simulink model "orbitCon"  (R2015b)
settings: Solver=VariableStepAuto  StartTime=0.0  StopTime=110376000  RelTol=1e-3
PreLoadFcn:
  | initialize
  | constants
values from neighbouring files (symbols this model uses):
  ini_pos = [6.6428e+3 * 10^3 ... (first row only)    [initialize.m]
  ini_vel = [  0.3023 * 10^3 ... (first row only)    [initialize.m]
settings Model: Creator=yyas16  LastModifiedBy=yyas16

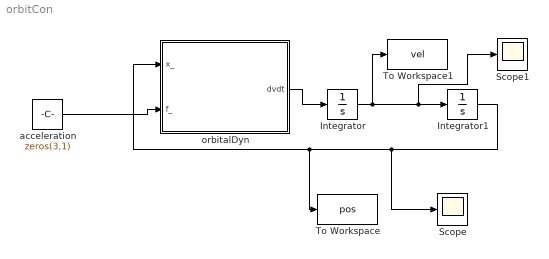
== system orbitCon ==
  Integrator : Integrator  InitialCondition=ini_vel
  Integrator1 : Integrator  InitialCondition=ini_pos
  Scope : Scope
  Scope1 : Scope
  To Workspace : ToWorkspace  VariableName=pos  SampleTime=-1
  To Workspace1 : ToWorkspace  VariableName=vel  SampleTime=-1
  acceleration : Constant  Value=zeros(3,1)
  orbitalDyn : MATLAB Function  TreatAsAtomicUnit=on
  wires:
  orbitalDyn/1(dvdt) -> Integrator/1
  Integrator/1 -> Scope1/1, Integrator1/1, To Workspace1/1
  Integrator1/1 -> Scope/1, To Workspace/1, orbitalDyn/1(x_)
  acceleration/1 -> orbitalDyn/2(f_)

== matlab function orbitCon/orbitalDyn ==
  data: x_ input; dvdt output; f_ input; GE parameter
function dvdt = orbitalDyn(x_, f_, GE)
%#codegen

% state variables
x  = x_(1);
y  = x_(2);
z  = x_(3);

r = sqrt(x^2 + y^2 + z^2); % Euclid norm
rVec = x_;

dvdt = -GE / r^3 .* rVec + f_;
